simulink model "model"  (R2024b)
settings: Solver=VariableStepAuto  StartTime=0.0  StopTime=10.0  RelTol=1e-3
libraries: simulink_extras x1
settings Model: Creator=HP  LastModifiedBy=HP

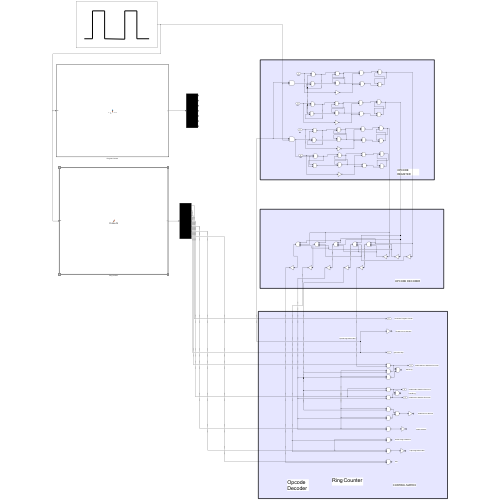
[thumbnail: Simulink's stored preview of the top-level diagram]
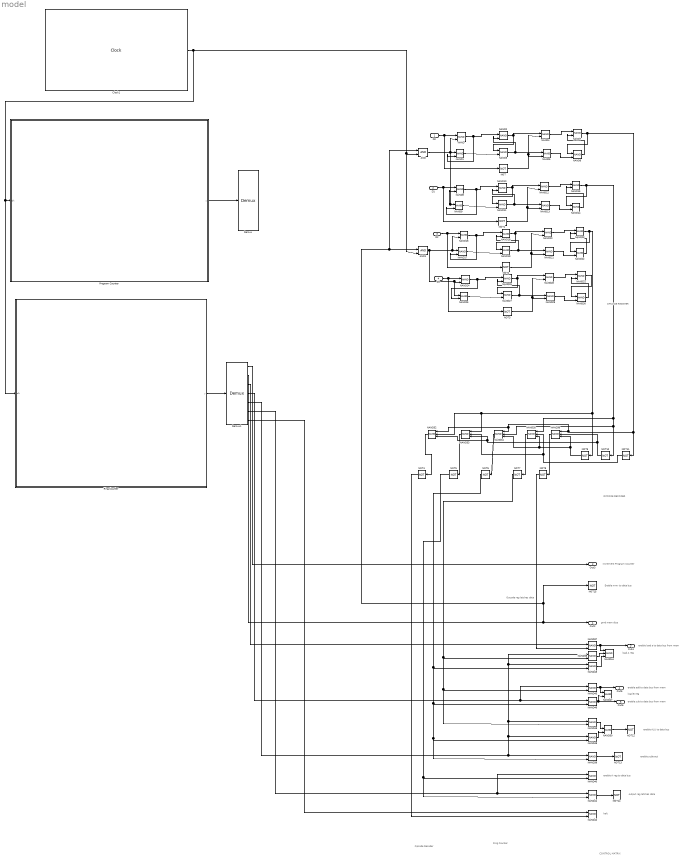
== system model ==
  note: CONTROL MATRIX
  note: OPCODE DECODER
  note: OPCODE
      | REGISTER
  note: halt
  note: enable subtract
  note: Increment Program Counter
  note: Opcode Decoder
  note: enable A reg to data bus
  note: enable sub to data bus from mem
  note: output reg latches data
  note: enable ALU to data bus
  note: enable add to data bus from mem
  note: load A reg
  note: Enable mmr to data bus
  note: enable load a to data bus from mem
  note: load B reg
  note: Opcode reg latches data
  note: Ring Counter
  note: grnd mem disp
  D0 : Inport
  D1 : Inport  Port=2
  D2 : Inport  Port=3
  D3 : Inport  Port=4
  AND : Logic  IconShape=distinctive  AllPortsSameDT=off  OutDataTypeStr=boolean
  AND1 : Logic  IconShape=distinctive  AllPortsSameDT=off  OutDataTypeStr=boolean
  Clock1 : simulink_extras/Flip Flops/Clock  period=2
  Demux : Demux  Outputs=7
  Demux1 : Demux  Outputs=7
  NAND{,1..31,37..43,45..50} (45 alike) : Logic  Operator=NAND  IconShape=distinctive  AllPortsSameDT=off  OutDataTypeStr=boolean
  NAND{32..36,44} (6 alike) : Logic  Operator=NAND  Inputs=3  IconShape=distinctive  AllPortsSameDT=off  OutDataTypeStr=boolean
  NOT{,1..15} (16 alike) : Logic  Operator=NOT  IconShape=distinctive  AllPortsSameDT=off  OutDataTypeStr=boolean
  Program Counter : MATLAB Function  TreatAsAtomicUnit=on
  Ring Counter : MATLAB Function  TreatAsAtomicUnit=on
  Out2 : Outport
  Out3 : Outport  Port=2
  Out4 : Outport  Port=3
  Out5 : Outport  Port=4
  Out6 : Outport  Port=5
  wires:
  Program Counter/1(y) -> Demux/1
  Ring Counter/1(y) -> Demux1/1
  NAND30/1 -> NAND31/2
  NOT1/1 -> NAND13/2, NAND12/2
  NAND28/1 -> NAND31/1
  NAND24/1 -> NAND25/2, NAND26/1
  NAND1/1 -> NAND3/2
  NAND5/1 -> NAND6/2
  NAND14/1 -> NAND15/2
  D2/1 -> NOT2/1, NAND16/1
  NAND19/1 -> NAND21/1, NAND18/2
  D1/1 -> NOT1/1, NAND8/1
  NAND13/1 -> NAND14/2
  NOT/1 -> NAND5/2, NAND4/2
  NOT2/1 -> NAND21/2, NAND20/2
  NAND6/1 -> NAND7/2
  NAND11/1 -> NAND13/1, NAND10/2
  NAND17/1 -> NAND19/2
  NAND10/1 -> NAND11/1, NAND12/1
  NAND/1 -> NAND1/2, NAND2/1
  NAND18/1 -> NAND20/1, NAND19/1
  NAND21/1 -> NAND22/2
  NAND26/1 -> NAND27/1, NAND28/1
  Clock1/1 -> AND1/2, AND/2, Ring Counter/1(clk), Program Counter/1(clk)
  NAND12/1 -> NAND15/1
  D3/1 -> NOT3/1, NAND24/1
  NAND9/1 -> NAND11/2
  NAND31/1 -> NAND30/1
  NAND29/1 -> NAND30/2
  NAND25/1 -> NAND27/2
  NAND3/1 -> NAND5/1, NAND2/2
  NAND22/1 -> NAND23/2
  D0/1 -> NOT/1, NAND/1
  AND1/1 -> NAND17/1, NAND16/2, NAND25/1, NAND24/2
  NAND20/1 -> NAND23/1
  NAND8/1 -> NAND9/2, NAND10/1
  NAND16/1 -> NAND17/2, NAND18/1
  AND/1 -> NAND8/2, NAND9/1, NAND1/1, NAND/2
  Demux1/2 -> Out2/1, AND1/1, AND/1, NOT15/1
  NAND4/1 -> NAND7/1
  NOT3/1 -> NAND29/2, NAND28/2
  NAND2/1 -> NAND3/1, NAND4/1
  NAND27/1 -> NAND29/1, NAND26/2
  NOT10/1 -> NAND32/3, NAND33/3, NAND36/2
  NOT11/1 -> NAND33/2, NAND35/2
  NAND33/1 -> NOT5/1
  NAND35/1 -> NOT7/1
  NAND7/1 -> NOT11/1, NAND32/1, NAND34/1, NAND36/1, NAND6/1
  NAND36/1 -> NOT8/1
  NAND34/1 -> NOT6/1
  NAND23/1 -> NAND32/2, NAND33/1, NOT9/1, NAND22/1
  NAND32/1 -> NOT4/1
  NAND15/1 -> NAND34/2, NOT10/1, NAND35/1, NAND14/1
  NOT9/1 -> NAND34/3, NAND35/3, NAND36/3
  NOT4/1 -> NAND42/2
  NAND37/1 -> Out4/1, NAND44/1
  NOT5/1 -> NAND41/2, NAND40/2
  NAND38/1 -> NAND44/2
  Demux1/5 -> NAND49/1, NAND48/1, NAND43/1, NAND38/1, NAND39/1
  NAND39/1 -> NOT13/1
  NAND46/1 -> Out6/1, NAND47/2
  NAND41/1 -> NOT14/1
  Demux1/4 -> NAND45/1, NAND46/1
  NAND50/1 -> NOT12/1
  Demux1/3 -> NAND37/1
  NOT7/1 -> NAND48/2, NAND45/2, NAND38/2
  NAND45/1 -> NAND47/1, Out5/1
  NAND49/1 -> NAND50/2
  NAND43/1 -> NAND44/3
  NAND48/1 -> NAND50/1
  NOT8/1 -> NAND37/2
  Demux1/6 -> NAND40/1, NAND41/1
  Demux1/1 -> Out3/1
  NOT6/1 -> NAND39/2, NAND49/2, NAND46/2, NAND43/2
  Demux1/7 -> NAND42/1

== matlab function model/Program Counter ==
  data: y output; clk input
function y = ring_counter(clk)
% 7-bit Ring Counter
persistent state
if isempty(state)
    state = [1 0 0 0 0 0 0]; % Initial state
end

if clk == 1
    state = circshift(state, [0 1]); % Shift right
end

y = state;

== matlab function model/Ring Counter ==
  data: y output; clk input
function y = ring_counter(clk)
% 7-bit Ring Counter
persistent state
if isempty(state)
    state = [1 0 0 0 0 0 0]; % Initial state
end

if clk == 1
    state = circshift(state, [0 1]); % Shift right
end

y = state;
